simulink model "Australian14gen_following_inertia"  (R2017b)
settings: Solver=ode23tb  StartTime=0.0  StopTime=30  FixedStep=1e-3  RelTol=1e-5  AbsTol=1e-3  EnableMultiTasking=on
PreLoadFcn:
  | dataaustralian14gen
values from neighbouring files (symbols this model uses):
  alpha = -sys.follin.opt.alpha*1e8    [main_following.m]    (also in optimgains.mat = [-2447350365.29 -12566370614.4 -12566370614.4 -11730281347.7)
  bus_v = [ 101	15 ... (first row only)    [dataaustralian14gen.m]
  comp = [ 1	211	0	0 ... (first row only)    [dataaustralian14gen.m]
  dist = sys.follin.dist    [main_following.m]    (also in main_forming.m = sys.formin.dist)
  Exc = [ 101	0	 200	0.1	    13.25  2.5	 0	0       0       0       0       0 ... (first row only)    [dataaustralian14gen.m]
  FH = 13    [dataaustralian14gen.m]
  FI = 1    [dataaustralian14gen.m]
  FL = .1    (= 0.1)    [dataaustralian14gen.m]
  G_data = [ 101	333.3	15	3.6	0.14	1.1	0.65	0.25	8.5     0.25	0.05	0       0       0.25	0.2 	0 ... (first row only)    [dataaustralian14gen.m]
  KH = 120    [dataaustralian14gen.m]
  KI = 10    [dataaustralian14gen.m]
  KL = 10    [dataaustralian14gen.m]
  line = [ 102	217	0.0084	0.0667	0.817	330	1 ... (first row only)    [dataaustralian14gen.m]
  load_mag = load_case4    [dataaustralian14gen.m]
  p = p_case4    [dataaustralian14gen.m]
  PLL_Ki = 2    [dataaustralian14gen.m]
  PLL_Kp = 500    [dataaustralian14gen.m]
  PSSMODEL = 1    [dataaustralian14gen.m]
  trans = [ 1	101	102	15	330	333.3	12	12 ... (first row only)    [dataaustralian14gen.m]
undefined symbols (not defined in the file or in its folder): D1, Delta, sys
libraries: powerlib x353, Library x30, powerlib_meascontrol x15, sps_avr x10, powerlib_extras x4
(part 4 of 4)

== system Australian14gen_following_inertia/VI403 ==
  Constant : Constant  Value=0
  Gain : Gain  Gain=-1
  Mux : Mux  Inputs=2
  Mux1 : Mux  Inputs=2
  PLL : Library/PLL  Kp=PLL_Kp  Ki=PLL_Ki  theta0=29.6583
  "Power (3ph, Phasor)" : powerlib_meascontrol/Measurements/Power (3ph, Phasor)
      settings: SourceProductName=Simscape Power Systems  SourceProductBaseCode=PS
  Scope : Scope
  Three-Phase V-I Measurement : powerlib/Measurements/Three-Phase V-I Measurement  VoltageMeasurement=phase-to-ground  SetLabelV=off  LabelV=Vabc  Vpu=off  VpuLL=off  CurrentMeasurement=yes  SetLabelI=off  LabelI=Iabc  Ipu=off  Pbase=100e6  Vbase=500e3  OutputType=Complex  PhasorSimulation=on  PSBequivalent=0
  dP102_vi : Library/dP102_vi  d=alpha(10)  m=alpha(25)
  virtin : powerlib/Elements/Three-Phase Dynamic Load  NominalVoltage=[ 20e3 50 ]  ActiveReactivePowers=[0 0]  PositiveSequence=[0.999418 29.6583]  ExternalControl=on  NpNq="[0  0]"  TimeConstants="[0  0  0  0]"  MinimumVoltage=0.01  Tfilter=1e-1  LoadFlowParameters=[4 50000000 0 0 25000000]
      settings: SourceProductName=Simscape Power Systems  SourceProductBaseCode=PS
  A : PMIOPort  Port=1  Side=Right
  B : PMIOPort  Port=2  Side=Right
  C : PMIOPort  Port=3  Side=Right
  tag scope: P403=global, Q403=global, w403=global
  wires:
  Mux/1 -> Gain/1
  Gain/1 -> virtin/1
  Constant/1 -> Mux/2
  dP102_vi/1 -> Mux/1
  [Vabc_B403] -> PLL/1
  PLL/1 -> Mux1/1, dP102_vi/1
  Mux1/1 -> [w403]
  PLL/2 -> Mux1/2, dP102_vi/2
  PLL/3 -> Scope/1
  "Power (3ph, Phasor)"/1 -> [P403]
  Three-Phase V-I Measurement/1 -> "Power (3ph, Phasor)"/1
  Three-Phase V-I Measurement/2 -> "Power (3ph, Phasor)"/2
  "Power (3ph, Phasor)"/2 -> [Q403]
  connections:
  B/RConn1 -- Three-Phase V-I Measurement/RConn2
  A/RConn1 -- Three-Phase V-I Measurement/RConn1
  C/RConn1 -- Three-Phase V-I Measurement/RConn3
  virtin/LConn1 -- Three-Phase V-I Measurement/LConn1
  virtin/LConn3 -- Three-Phase V-I Measurement/LConn3
  virtin/LConn2 -- Three-Phase V-I Measurement/LConn2

== system Australian14gen_following_inertia/VI405 ==
  Constant : Constant  Value=0
  Gain : Gain  Gain=-1
  Mux : Mux  Inputs=2
  Mux1 : Mux  Inputs=2
  PLL : Library/PLL  Kp=PLL_Kp  Ki=PLL_Ki  theta0=16.7314
  "Power (3ph, Phasor)" : powerlib_meascontrol/Measurements/Power (3ph, Phasor)
      settings: SourceProductName=Simscape Power Systems  SourceProductBaseCode=PS
  Three-Phase V-I Measurement : powerlib/Measurements/Three-Phase V-I Measurement  VoltageMeasurement=phase-to-ground  SetLabelV=off  LabelV=Vabc  Vpu=off  VpuLL=off  CurrentMeasurement=yes  SetLabelI=off  LabelI=Iabc  Ipu=off  Pbase=100e6  Vbase=500e3  OutputType=Complex  PhasorSimulation=on  PSBequivalent=0
  dP102_vi : Library/dP102_vi  d=alpha(11)  m=alpha(26)
  virtin : powerlib/Elements/Three-Phase Dynamic Load  NominalVoltage=[20e3 50 ]  ActiveReactivePowers=[0 0]  PositiveSequence=[1.00896 16.7314]  ExternalControl=on  NpNq="[0  0]"  TimeConstants="[0  0  0  0]"  MinimumVoltage=0.01  Tfilter=1e-1  LoadFlowParameters=[4 50000000 0 0 25000000]
      settings: SourceProductName=Simscape Power Systems  SourceProductBaseCode=PS
  A : PMIOPort  Port=1  Side=Right
  B : PMIOPort  Port=2  Side=Right
  C : PMIOPort  Port=3  Side=Right
  tag scope: P405=global, Q405=global, w405=global
  wires:
  Mux/1 -> Gain/1
  Gain/1 -> virtin/1
  Constant/1 -> Mux/2
  dP102_vi/1 -> Mux/1
  [Vabc_B405_vi] -> PLL/1
  PLL/1 -> Mux1/1, dP102_vi/1
  Mux1/1 -> [w405]
  PLL/2 -> Mux1/2, dP102_vi/2
  "Power (3ph, Phasor)"/1 -> [P405]
  Three-Phase V-I Measurement/1 -> "Power (3ph, Phasor)"/1
  Three-Phase V-I Measurement/2 -> "Power (3ph, Phasor)"/2
  "Power (3ph, Phasor)"/2 -> [Q405]
  connections:
  B/RConn1 -- Three-Phase V-I Measurement/RConn2
  A/RConn1 -- Three-Phase V-I Measurement/RConn1
  C/RConn1 -- Three-Phase V-I Measurement/RConn3
  virtin/LConn1 -- Three-Phase V-I Measurement/LConn1
  virtin/LConn3 -- Three-Phase V-I Measurement/LConn3
  virtin/LConn2 -- Three-Phase V-I Measurement/LConn2

== system Australian14gen_following_inertia/VI410 ==
  Constant : Constant  Value=0
  Gain : Gain  Gain=-1
  Mux : Mux  Inputs=2
  Mux1 : Mux  Inputs=2
  PLL : Library/PLL  Kp=PLL_Kp  Ki=PLL_Ki  theta0=8.97655
  "Power (3ph, Phasor)" : powerlib_meascontrol/Measurements/Power (3ph, Phasor)
      settings: SourceProductName=Simscape Power Systems  SourceProductBaseCode=PS
  Three-Phase V-I Measurement : powerlib/Measurements/Three-Phase V-I Measurement  VoltageMeasurement=phase-to-ground  SetLabelV=off  LabelV=Vabc  Vpu=off  VpuLL=off  CurrentMeasurement=yes  SetLabelI=off  LabelI=Iabc  Ipu=off  Pbase=100e6  Vbase=500e3  OutputType=Complex  PhasorSimulation=on  PSBequivalent=0
  dP102_vi : Library/dP102_vi  d=alpha(12)  m=alpha(27)
  dw : Scope
  theta : Scope
  virtin : powerlib/Elements/Three-Phase Dynamic Load  NominalVoltage=[ 20e3 50 ]  ActiveReactivePowers=[0 0]  PositiveSequence=[1.01728 8.97655]  ExternalControl=on  NpNq="[0  0]"  TimeConstants="[0  0  0  0]"  MinimumVoltage=0.01  Tfilter=1e-1  LoadFlowParameters=[4 50000000 0 0 25000000]
      settings: SourceProductName=Simscape Power Systems  SourceProductBaseCode=PS
  w : Scope
  A : PMIOPort  Port=1  Side=Right
  B : PMIOPort  Port=2  Side=Right
  C : PMIOPort  Port=3  Side=Right
  tag scope: P410=global, Q410=global, w410=global
  wires:
  Mux/1 -> Gain/1
  Gain/1 -> virtin/1
  Constant/1 -> Mux/2
  dP102_vi/1 -> Mux/1
  [Vabc_B410_vi] -> PLL/1
  Mux1/1 -> [w410]
  PLL/1 -> w/1, Mux1/1, dP102_vi/1
  PLL/2 -> dw/1, Mux1/2, dP102_vi/2
  PLL/3 -> theta/1
  Three-Phase V-I Measurement/1 -> "Power (3ph, Phasor)"/1
  Three-Phase V-I Measurement/2 -> "Power (3ph, Phasor)"/2
  "Power (3ph, Phasor)"/1 -> [P410]
  "Power (3ph, Phasor)"/2 -> [Q410]
  connections:
  Three-Phase V-I Measurement/RConn1 -- A/RConn1
  B/RConn1 -- Three-Phase V-I Measurement/RConn2
  Three-Phase V-I Measurement/RConn3 -- C/RConn1
  virtin/LConn1 -- Three-Phase V-I Measurement/LConn1
  virtin/LConn2 -- Three-Phase V-I Measurement/LConn2
  virtin/LConn3 -- Three-Phase V-I Measurement/LConn3

== system Australian14gen_following_inertia/VI502 ==
  Constant : Constant  Value=0
  Gain : Gain  Gain=-1
  Mux : Mux  Inputs=2
  Mux1 : Mux  Inputs=2
  PLL : Library/PLL  Kp=PLL_Kp  Ki=PLL_Ki  theta0=-2.58144
  "Power (3ph, Phasor)" : powerlib_meascontrol/Measurements/Power (3ph, Phasor)
      settings: SourceProductName=Simscape Power Systems  SourceProductBaseCode=PS
  Three-Phase V-I Measurement : powerlib/Measurements/Three-Phase V-I Measurement  VoltageMeasurement=phase-to-ground  SetLabelV=off  LabelV=Vabc  Vpu=off  VpuLL=off  CurrentMeasurement=yes  SetLabelI=off  LabelI=Iabc  Ipu=off  Pbase=100e6  Vbase=500e3  OutputType=Complex  PhasorSimulation=on  PSBequivalent=0
  dP102_vi : Library/dP102_vi  d=alpha(13)  m=alpha(28)
  virtin : powerlib/Elements/Three-Phase Dynamic Load  NominalVoltage=[ 20e3 50 ]  ActiveReactivePowers=[0 0]  PositiveSequence=[0.0544568 -2.58144]  ExternalControl=on  NpNq="[0  0]"  TimeConstants="[0  0  0  0]"  MinimumVoltage=0.01  Tfilter=1e-1  LoadFlowParameters=[4 50000000 0 0 25000000]
      settings: SourceProductName=Simscape Power Systems  SourceProductBaseCode=PS
  A : PMIOPort  Port=1  Side=Right
  B : PMIOPort  Port=2  Side=Right
  C : PMIOPort  Port=3  Side=Right
  tag scope: P502=global, Q502=global, w502=global
  wires:
  Mux/1 -> Gain/1
  Gain/1 -> virtin/1
  Constant/1 -> Mux/2
  dP102_vi/1 -> Mux/1
  [Vabc_B502_vi] -> PLL/1
  PLL/1 -> dP102_vi/1, Mux1/1
  Mux1/1 -> [w502]
  PLL/2 -> Mux1/2, dP102_vi/2
  "Power (3ph, Phasor)"/1 -> [P502]
  Three-Phase V-I Measurement/1 -> "Power (3ph, Phasor)"/1
  "Power (3ph, Phasor)"/2 -> [Q502]
  Three-Phase V-I Measurement/2 -> "Power (3ph, Phasor)"/2
  connections:
  virtin/LConn1 -- Three-Phase V-I Measurement/LConn1
  C/RConn1 -- Three-Phase V-I Measurement/RConn3
  virtin/LConn3 -- Three-Phase V-I Measurement/LConn3
  B/RConn1 -- Three-Phase V-I Measurement/RConn2
  virtin/LConn2 -- Three-Phase V-I Measurement/LConn2
  A/RConn1 -- Three-Phase V-I Measurement/RConn1

== system Australian14gen_following_inertia/VI504 ==
  Constant : Constant  Value=0
  Gain : Gain  Gain=-1
  Mux : Mux  Inputs=2
  Mux1 : Mux  Inputs=2
  PLL : Library/PLL  Kp=PLL_Kp  Ki=PLL_Ki  theta0=-12.1555
  "Power (3ph, Phasor)" : powerlib_meascontrol/Measurements/Power (3ph, Phasor)
      settings: SourceProductName=Simscape Power Systems  SourceProductBaseCode=PS
  Three-Phase V-I Measurement : powerlib/Measurements/Three-Phase V-I Measurement  VoltageMeasurement=phase-to-ground  SetLabelV=off  LabelV=Vabc  Vpu=off  VpuLL=off  CurrentMeasurement=yes  SetLabelI=off  LabelI=Iabc  Ipu=off  Pbase=100e6  Vbase=500e3  OutputType=Complex  PhasorSimulation=on  PSBequivalent=0
  dP102_vi : Library/dP102_vi  d=alpha(14)  m=alpha(29)
  virtin : powerlib/Elements/Three-Phase Dynamic Load  NominalVoltage=[ 20e3 50 ]  ActiveReactivePowers=[0 0]  PositiveSequence=[1.03954 -12.1555]  ExternalControl=on  NpNq="[0  0]"  TimeConstants="[0  0  0  0]"  MinimumVoltage=0.01  Tfilter=1e-1  LoadFlowParameters=[4 50000000 0 0 25000000]
      settings: SourceProductName=Simscape Power Systems  SourceProductBaseCode=PS
  A : PMIOPort  Port=1  Side=Right
  B : PMIOPort  Port=2  Side=Right
  C : PMIOPort  Port=3  Side=Right
  tag scope: P504=global, Q504=global, w504=global
  wires:
  Mux/1 -> Gain/1
  Gain/1 -> virtin/1
  Constant/1 -> Mux/2
  dP102_vi/1 -> Mux/1
  [Vabc_B504_vi] -> PLL/1
  PLL/1 -> Mux1/1, dP102_vi/1
  Mux1/1 -> [w504]
  PLL/2 -> Mux1/2, dP102_vi/2
  "Power (3ph, Phasor)"/1 -> [P504]
  Three-Phase V-I Measurement/1 -> "Power (3ph, Phasor)"/1
  "Power (3ph, Phasor)"/2 -> [Q504]
  Three-Phase V-I Measurement/2 -> "Power (3ph, Phasor)"/2
  connections:
  virtin/LConn1 -- Three-Phase V-I Measurement/LConn1
  C/RConn1 -- Three-Phase V-I Measurement/RConn3
  virtin/LConn3 -- Three-Phase V-I Measurement/LConn3
  B/RConn1 -- Three-Phase V-I Measurement/RConn2
  virtin/LConn2 -- Three-Phase V-I Measurement/LConn2
  A/RConn1 -- Three-Phase V-I Measurement/RConn1

== system Australian14gen_following_inertia/VI508 ==
  Constant : Constant  Value=0
  Gain : Gain  Gain=-1
  Mux : Mux  Inputs=2
  Mux1 : Mux  Inputs=2
  PLL : Library/PLL  Kp=PLL_Kp  Ki=PLL_Ki  theta0=-14.4633
  "Power (3ph, Phasor)" : powerlib_meascontrol/Measurements/Power (3ph, Phasor)
      settings: SourceProductName=Simscape Power Systems  SourceProductBaseCode=PS
  Three-Phase V-I Measurement : powerlib/Measurements/Three-Phase V-I Measurement  VoltageMeasurement=phase-to-ground  SetLabelV=off  LabelV=Vabc  Vpu=off  VpuLL=off  CurrentMeasurement=yes  SetLabelI=off  LabelI=Iabc  Ipu=off  Pbase=100e6  Vbase=500e3  OutputType=Complex  PhasorSimulation=on  PSBequivalent=0
  dP102_vi : Library/dP102_vi  d=alpha(15)  m=alpha(30)
  virtin : powerlib/Elements/Three-Phase Dynamic Load  NominalVoltage=[ 15e3 50 ]  ActiveReactivePowers=[0 0]  PositiveSequence=[1.00927 -14.4633]  ExternalControl=on  NpNq="[0  0]"  TimeConstants="[0  0  0  0]"  MinimumVoltage=0.01  Tfilter=1e-1  LoadFlowParameters=[4 50000000 0 0 25000000]
      settings: SourceProductName=Simscape Power Systems  SourceProductBaseCode=PS
  A : PMIOPort  Port=1  Side=Right
  B : PMIOPort  Port=2  Side=Right
  C : PMIOPort  Port=3  Side=Right
  tag scope: P508=global, Q508=global, w508=global
  wires:
  Mux/1 -> Gain/1
  Gain/1 -> virtin/1
  Constant/1 -> Mux/2
  dP102_vi/1 -> Mux/1
  [Vabc_B508_vi] -> PLL/1
  PLL/1 -> Mux1/1, dP102_vi/1
  Mux1/1 -> [w508]
  PLL/2 -> Mux1/2, dP102_vi/2
  "Power (3ph, Phasor)"/1 -> [P508]
  Three-Phase V-I Measurement/1 -> "Power (3ph, Phasor)"/1
  "Power (3ph, Phasor)"/2 -> [Q508]
  Three-Phase V-I Measurement/2 -> "Power (3ph, Phasor)"/2
  connections:
  virtin/LConn1 -- Three-Phase V-I Measurement/LConn1
  C/RConn1 -- Three-Phase V-I Measurement/RConn3
  virtin/LConn3 -- Three-Phase V-I Measurement/LConn3
  B/RConn1 -- Three-Phase V-I Measurement/RConn2
  virtin/LConn2 -- Three-Phase V-I Measurement/LConn2
  A/RConn1 -- Three-Phase V-I Measurement/RConn1
